simulink model "sim_sys2"  (R2013b)
settings: Solver=ode45  StartTime=0.0  StopTime=5000  RelTol=1e-3
undefined symbols (not defined in the file or in its folder): msdft_comb, resonator, sys_lib, twiddle_factors
libraries: xbsIndex_r4 x3996, casper_library_misc x310, xps_library x1
(part 2 of 46)

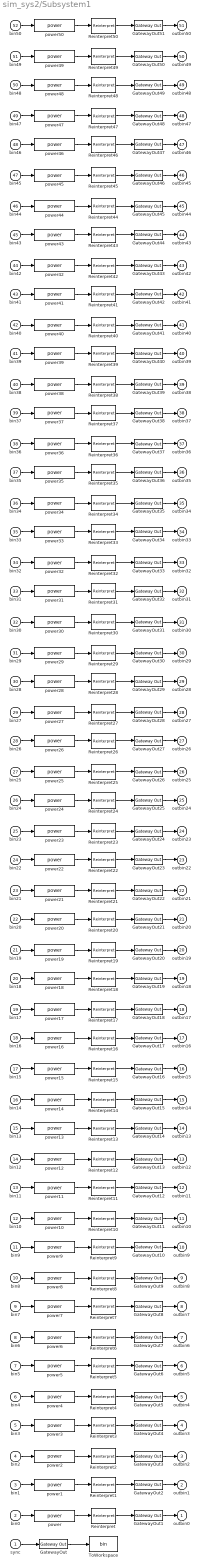
== system sim_sys2/Subsystem1 ==
  sync : Inport
  bin0 : Inport  Port=2
  bin1 : Inport  Port=3
  bin2 : Inport  Port=4
  bin3 : Inport  Port=5
  bin4 : Inport  Port=6
  bin5 : Inport  Port=7
  bin6 : Inport  Port=8
  bin7 : Inport  Port=9
  bin8 : Inport  Port=10
  bin9 : Inport  Port=11
  bin10 : Inport  Port=12
  bin11 : Inport  Port=13
  bin12 : Inport  Port=14
  bin13 : Inport  Port=15
  bin14 : Inport  Port=16
  bin15 : Inport  Port=17
  bin16 : Inport  Port=18
  bin17 : Inport  Port=19
  bin18 : Inport  Port=20
  bin19 : Inport  Port=21
  bin20 : Inport  Port=22
  bin21 : Inport  Port=23
  bin22 : Inport  Port=24
  bin23 : Inport  Port=25
  bin24 : Inport  Port=26
  bin25 : Inport  Port=27
  bin26 : Inport  Port=28
  bin27 : Inport  Port=29
  bin28 : Inport  Port=30
  bin29 : Inport  Port=31
  bin30 : Inport  Port=32
  bin31 : Inport  Port=33
  bin32 : Inport  Port=34
  bin33 : Inport  Port=35
  bin34 : Inport  Port=36
  bin35 : Inport  Port=37
  bin36 : Inport  Port=38
  bin37 : Inport  Port=39
  bin38 : Inport  Port=40
  bin39 : Inport  Port=41
  bin40 : Inport  Port=42
  bin41 : Inport  Port=43
  bin42 : Inport  Port=44
  bin43 : Inport  Port=45
  bin44 : Inport  Port=46
  bin45 : Inport  Port=47
  bin46 : Inport  Port=48
  bin47 : Inport  Port=49
  bin48 : Inport  Port=50
  bin49 : Inport  Port=51
  bin50 : Inport  Port=52
  GatewayOut{,1..51} (52 alike) : xbsIndex_r4/Gateway Out  inherit_from_input=on  hdl_port=on  timing_constraint=None  locs_specified=off  LOCs={}  UseAsDAC=off  DACChannel='1'  block_type=gatewayout
  Reinterpret{,1..50} (51 alike) : xbsIndex_r4/Reinterpret  force_arith_type=off  arith_type=Unsigned  force_bin_pt=on  bin_pt=0  block_type=reinterpret
  ToWorkspace : ToWorkspace  VariableName=bin  SampleTime=-1  SaveFormat=Timeseries
  power{,1..50} (51 alike) : casper_library_misc/power  BitWidth=40  add_latency=2  mult_latency=3
  outbin0 : Outport
  outbin1 : Outport  Port=2
  outbin2 : Outport  Port=3
  outbin3 : Outport  Port=4
  outbin4 : Outport  Port=5
  outbin5 : Outport  Port=6
  outbin6 : Outport  Port=7
  outbin7 : Outport  Port=8
  outbin8 : Outport  Port=9
  outbin9 : Outport  Port=10
  outbin10 : Outport  Port=11
  outbin11 : Outport  Port=12
  outbin12 : Outport  Port=13
  outbin13 : Outport  Port=14
  outbin14 : Outport  Port=15
  outbin15 : Outport  Port=16
  outbin16 : Outport  Port=17
  outbin17 : Outport  Port=18
  outbin18 : Outport  Port=19
  outbin19 : Outport  Port=20
  outbin20 : Outport  Port=21
  outbin21 : Outport  Port=22
  outbin22 : Outport  Port=23
  outbin23 : Outport  Port=24
  outbin24 : Outport  Port=25
  outbin25 : Outport  Port=26
  outbin26 : Outport  Port=27
  outbin27 : Outport  Port=28
  outbin28 : Outport  Port=29
  outbin29 : Outport  Port=30
  outbin30 : Outport  Port=31
  outbin31 : Outport  Port=32
  outbin32 : Outport  Port=33
  outbin33 : Outport  Port=34
  outbin34 : Outport  Port=35
  outbin35 : Outport  Port=36
  outbin36 : Outport  Port=37
  outbin37 : Outport  Port=38
  outbin38 : Outport  Port=39
  outbin39 : Outport  Port=40
  outbin40 : Outport  Port=41
  outbin41 : Outport  Port=42
  outbin42 : Outport  Port=43
  outbin43 : Outport  Port=44
  outbin44 : Outport  Port=45
  outbin45 : Outport  Port=46
  outbin46 : Outport  Port=47
  outbin47 : Outport  Port=48
  outbin48 : Outport  Port=49
  outbin49 : Outport  Port=50
  outbin50 : Outport  Port=51
  wires:
  GatewayOut51/1 -> outbin50/1
  Reinterpret50/1 -> GatewayOut51/1
  power50/1 -> Reinterpret50/1
  bin50/1 -> power50/1
  GatewayOut50/1 -> outbin49/1
  Reinterpret49/1 -> GatewayOut50/1
  power49/1 -> Reinterpret49/1
  bin49/1 -> power49/1
  GatewayOut49/1 -> outbin48/1
  Reinterpret48/1 -> GatewayOut49/1
  power48/1 -> Reinterpret48/1
  bin48/1 -> power48/1
  GatewayOut48/1 -> outbin47/1
  Reinterpret47/1 -> GatewayOut48/1
  power47/1 -> Reinterpret47/1
  bin47/1 -> power47/1
  GatewayOut47/1 -> outbin46/1
  Reinterpret46/1 -> GatewayOut47/1
  power46/1 -> Reinterpret46/1
  bin46/1 -> power46/1
  GatewayOut46/1 -> outbin45/1
  Reinterpret45/1 -> GatewayOut46/1
  power45/1 -> Reinterpret45/1
  bin45/1 -> power45/1
  GatewayOut45/1 -> outbin44/1
  Reinterpret44/1 -> GatewayOut45/1
  power44/1 -> Reinterpret44/1
  bin44/1 -> power44/1
  GatewayOut44/1 -> outbin43/1
  Reinterpret43/1 -> GatewayOut44/1
  power43/1 -> Reinterpret43/1
  bin43/1 -> power43/1
  GatewayOut43/1 -> outbin42/1
  Reinterpret42/1 -> GatewayOut43/1
  power42/1 -> Reinterpret42/1
  bin42/1 -> power42/1
  GatewayOut42/1 -> outbin41/1
  Reinterpret41/1 -> GatewayOut42/1
  power41/1 -> Reinterpret41/1
  bin41/1 -> power41/1
  GatewayOut41/1 -> outbin40/1
  Reinterpret40/1 -> GatewayOut41/1
  power40/1 -> Reinterpret40/1
  bin40/1 -> power40/1
  GatewayOut40/1 -> outbin39/1
  Reinterpret39/1 -> GatewayOut40/1
  power39/1 -> Reinterpret39/1
  bin39/1 -> power39/1
  GatewayOut39/1 -> outbin38/1
  Reinterpret38/1 -> GatewayOut39/1
  power38/1 -> Reinterpret38/1
  bin38/1 -> power38/1
  GatewayOut38/1 -> outbin37/1
  Reinterpret37/1 -> GatewayOut38/1
  power37/1 -> Reinterpret37/1
  bin37/1 -> power37/1
  GatewayOut37/1 -> outbin36/1
  Reinterpret36/1 -> GatewayOut37/1
  power36/1 -> Reinterpret36/1
  bin36/1 -> power36/1
  GatewayOut36/1 -> outbin35/1
  Reinterpret35/1 -> GatewayOut36/1
  power35/1 -> Reinterpret35/1
  bin35/1 -> power35/1
  GatewayOut35/1 -> outbin34/1
  Reinterpret34/1 -> GatewayOut35/1
  power34/1 -> Reinterpret34/1
  bin34/1 -> power34/1
  GatewayOut34/1 -> outbin33/1
  Reinterpret33/1 -> GatewayOut34/1
  power33/1 -> Reinterpret33/1
  bin33/1 -> power33/1
  GatewayOut33/1 -> outbin32/1
  Reinterpret32/1 -> GatewayOut33/1
  power32/1 -> Reinterpret32/1
  bin32/1 -> power32/1
  GatewayOut32/1 -> outbin31/1
  Reinterpret31/1 -> GatewayOut32/1
  power31/1 -> Reinterpret31/1
  bin31/1 -> power31/1
  GatewayOut31/1 -> outbin30/1
  Reinterpret30/1 -> GatewayOut31/1
  power30/1 -> Reinterpret30/1
  bin30/1 -> power30/1
  GatewayOut30/1 -> outbin29/1
  Reinterpret29/1 -> GatewayOut30/1
  power29/1 -> Reinterpret29/1
  bin29/1 -> power29/1
  GatewayOut29/1 -> outbin28/1
  Reinterpret28/1 -> GatewayOut29/1
  power28/1 -> Reinterpret28/1
  bin28/1 -> power28/1
  GatewayOut28/1 -> outbin27/1
  Reinterpret27/1 -> GatewayOut28/1
  power27/1 -> Reinterpret27/1
  bin27/1 -> power27/1
  GatewayOut27/1 -> outbin26/1
  Reinterpret26/1 -> GatewayOut27/1
  power26/1 -> Reinterpret26/1
  bin26/1 -> power26/1
  GatewayOut26/1 -> outbin25/1
  Reinterpret25/1 -> GatewayOut26/1
  power25/1 -> Reinterpret25/1
  bin25/1 -> power25/1
  GatewayOut25/1 -> outbin24/1
  Reinterpret24/1 -> GatewayOut25/1
  power24/1 -> Reinterpret24/1
  bin24/1 -> power24/1
  GatewayOut24/1 -> outbin23/1
  Reinterpret23/1 -> GatewayOut24/1
  power23/1 -> Reinterpret23/1
  bin23/1 -> power23/1
  GatewayOut23/1 -> outbin22/1
  Reinterpret22/1 -> GatewayOut23/1
  power22/1 -> Reinterpret22/1
  bin22/1 -> power22/1
  GatewayOut22/1 -> outbin21/1
  Reinterpret21/1 -> GatewayOut22/1
  power21/1 -> Reinterpret21/1
  bin21/1 -> power21/1
  GatewayOut21/1 -> outbin20/1
  Reinterpret20/1 -> GatewayOut21/1
  power20/1 -> Reinterpret20/1
  bin20/1 -> power20/1
  GatewayOut20/1 -> outbin19/1
  Reinterpret19/1 -> GatewayOut20/1
  power19/1 -> Reinterpret19/1
  bin19/1 -> power19/1
  GatewayOut19/1 -> outbin18/1
  Reinterpret18/1 -> GatewayOut19/1
  power18/1 -> Reinterpret18/1
  bin18/1 -> power18/1
  GatewayOut18/1 -> outbin17/1
  Reinterpret17/1 -> GatewayOut18/1
  power17/1 -> Reinterpret17/1
  bin17/1 -> power17/1
  GatewayOut17/1 -> outbin16/1
  Reinterpret16/1 -> GatewayOut17/1
  power16/1 -> Reinterpret16/1
  bin16/1 -> power16/1
  GatewayOut16/1 -> outbin15/1
  Reinterpret15/1 -> GatewayOut16/1
  power15/1 -> Reinterpret15/1
  bin15/1 -> power15/1
  GatewayOut15/1 -> outbin14/1
  Reinterpret14/1 -> GatewayOut15/1
  power14/1 -> Reinterpret14/1
  bin14/1 -> power14/1
  GatewayOut14/1 -> outbin13/1
  Reinterpret13/1 -> GatewayOut14/1
  power13/1 -> Reinterpret13/1
  bin13/1 -> power13/1
  GatewayOut13/1 -> outbin12/1
  Reinterpret12/1 -> GatewayOut13/1
  power12/1 -> Reinterpret12/1
  bin12/1 -> power12/1
  GatewayOut12/1 -> outbin11/1
  Reinterpret11/1 -> GatewayOut12/1
  power11/1 -> Reinterpret11/1
  bin11/1 -> power11/1
  GatewayOut11/1 -> outbin10/1
  Reinterpret10/1 -> GatewayOut11/1
  power10/1 -> Reinterpret10/1
  bin10/1 -> power10/1
  GatewayOut10/1 -> outbin9/1
  Reinterpret9/1 -> GatewayOut10/1
  power9/1 -> Reinterpret9/1
  bin9/1 -> power9/1
  GatewayOut9/1 -> outbin8/1
  Reinterpret8/1 -> GatewayOut9/1
  power8/1 -> Reinterpret8/1
  bin8/1 -> power8/1
  GatewayOut8/1 -> outbin7/1
  Reinterpret7/1 -> GatewayOut8/1
  power7/1 -> Reinterpret7/1
  bin7/1 -> power7/1
  GatewayOut7/1 -> outbin6/1
  Reinterpret6/1 -> GatewayOut7/1
  power6/1 -> Reinterpret6/1
  bin6/1 -> power6/1
  GatewayOut6/1 -> outbin5/1
  Reinterpret5/1 -> GatewayOut6/1
  power5/1 -> Reinterpret5/1
  bin5/1 -> power5/1
  GatewayOut5/1 -> outbin4/1
  Reinterpret4/1 -> GatewayOut5/1
  power4/1 -> Reinterpret4/1
  bin4/1 -> power4/1
  GatewayOut4/1 -> outbin3/1
  Reinterpret3/1 -> GatewayOut4/1
  power3/1 -> Reinterpret3/1
  bin3/1 -> power3/1
  GatewayOut3/1 -> outbin2/1
  Reinterpret2/1 -> GatewayOut3/1
  power2/1 -> Reinterpret2/1
  bin2/1 -> power2/1
  GatewayOut2/1 -> outbin1/1
  Reinterpret1/1 -> GatewayOut2/1
  power1/1 -> Reinterpret1/1
  bin1/1 -> power1/1
  GatewayOut1/1 -> outbin0/1
  Reinterpret/1 -> GatewayOut1/1
  power/1 -> Reinterpret/1
  bin0/1 -> power/1
  GatewayOut/1 -> ToWorkspace/1
  sync/1 -> GatewayOut/1

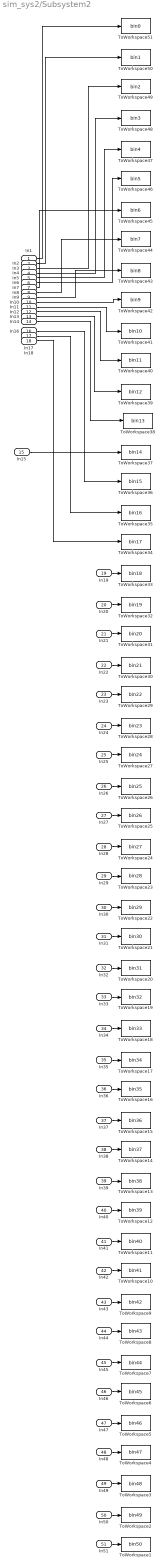
== system sim_sys2/Subsystem2 ==
  In1 : Inport
  In2 : Inport  Port=2
  In3 : Inport  Port=3
  In4 : Inport  Port=4
  In5 : Inport  Port=5
  In6 : Inport  Port=6
  In7 : Inport  Port=7
  In8 : Inport  Port=8
  In9 : Inport  Port=9
  In10 : Inport  Port=10
  In11 : Inport  Port=11
  In12 : Inport  Port=12
  In13 : Inport  Port=13
  In14 : Inport  Port=14
  In15 : Inport  Port=15
  In16 : Inport  Port=16
  In17 : Inport  Port=17
  In18 : Inport  Port=18
  In19 : Inport  Port=19
  In20 : Inport  Port=20
  In21 : Inport  Port=21
  In22 : Inport  Port=22
  In23 : Inport  Port=23
  In24 : Inport  Port=24
  In25 : Inport  Port=25
  In26 : Inport  Port=26
  In27 : Inport  Port=27
  In28 : Inport  Port=28
  In29 : Inport  Port=29
  In30 : Inport  Port=30
  In31 : Inport  Port=31
  In32 : Inport  Port=32
  In33 : Inport  Port=33
  In34 : Inport  Port=34
  In35 : Inport  Port=35
  In36 : Inport  Port=36
  In37 : Inport  Port=37
  In38 : Inport  Port=38
  In39 : Inport  Port=39
  In40 : Inport  Port=40
  In41 : Inport  Port=41
  In42 : Inport  Port=42
  In43 : Inport  Port=43
  In44 : Inport  Port=44
  In45 : Inport  Port=45
  In46 : Inport  Port=46
  In47 : Inport  Port=47
  In48 : Inport  Port=48
  In49 : Inport  Port=49
  In50 : Inport  Port=50
  In51 : Inport  Port=51
  ToWorkspace1 : ToWorkspace  VariableName=bin50  SampleTime=-1  SaveFormat=Timeseries
  ToWorkspace10 : ToWorkspace  VariableName=bin41  SampleTime=-1  SaveFormat=Timeseries
  ToWorkspace11 : ToWorkspace  VariableName=bin40  SampleTime=-1  SaveFormat=Timeseries
  ToWorkspace12 : ToWorkspace  VariableName=bin39  SampleTime=-1  SaveFormat=Timeseries
  ToWorkspace13 : ToWorkspace  VariableName=bin38  SampleTime=-1  SaveFormat=Timeseries
  ToWorkspace14 : ToWorkspace  VariableName=bin37  SampleTime=-1  SaveFormat=Timeseries
  ToWorkspace15 : ToWorkspace  VariableName=bin36  SampleTime=-1  SaveFormat=Timeseries
  ToWorkspace16 : ToWorkspace  VariableName=bin35  SampleTime=-1  SaveFormat=Timeseries
  ToWorkspace17 : ToWorkspace  VariableName=bin34  SampleTime=-1  SaveFormat=Timeseries
  ToWorkspace18 : ToWorkspace  VariableName=bin33  SampleTime=-1  SaveFormat=Timeseries
  ToWorkspace19 : ToWorkspace  VariableName=bin32  SampleTime=-1  SaveFormat=Timeseries
  ToWorkspace2 : ToWorkspace  VariableName=bin49  SampleTime=-1  SaveFormat=Timeseries
  ToWorkspace20 : ToWorkspace  VariableName=bin31  SampleTime=-1  SaveFormat=Timeseries
  ToWorkspace21 : ToWorkspace  VariableName=bin30  SampleTime=-1  SaveFormat=Timeseries
  ToWorkspace22 : ToWorkspace  VariableName=bin29  SampleTime=-1  SaveFormat=Timeseries
  ToWorkspace23 : ToWorkspace  VariableName=bin28  SampleTime=-1  SaveFormat=Timeseries
  ToWorkspace24 : ToWorkspace  VariableName=bin27  SampleTime=-1  SaveFormat=Timeseries
  ToWorkspace25 : ToWorkspace  VariableName=bin26  SampleTime=-1  SaveFormat=Timeseries
  ToWorkspace26 : ToWorkspace  VariableName=bin25  SampleTime=-1  SaveFormat=Timeseries
  ToWorkspace27 : ToWorkspace  VariableName=bin24  SampleTime=-1  SaveFormat=Timeseries
  ToWorkspace28 : ToWorkspace  VariableName=bin23  SampleTime=-1  SaveFormat=Timeseries
  ToWorkspace29 : ToWorkspace  VariableName=bin22  SampleTime=-1  SaveFormat=Timeseries
  ToWorkspace3 : ToWorkspace  VariableName=bin48  SampleTime=-1  SaveFormat=Timeseries
  ToWorkspace30 : ToWorkspace  VariableName=bin21  SampleTime=-1  SaveFormat=Timeseries
  ToWorkspace31 : ToWorkspace  VariableName=bin20  SampleTime=-1  SaveFormat=Timeseries
  ToWorkspace32 : ToWorkspace  VariableName=bin19  SampleTime=-1  SaveFormat=Timeseries
  ToWorkspace33 : ToWorkspace  VariableName=bin18  SampleTime=-1  SaveFormat=Timeseries
  ToWorkspace34 : ToWorkspace  VariableName=bin17  SampleTime=-1  SaveFormat=Timeseries
  ToWorkspace35 : ToWorkspace  VariableName=bin16  SampleTime=-1  SaveFormat=Timeseries
  ToWorkspace36 : ToWorkspace  VariableName=bin15  SampleTime=-1  SaveFormat=Timeseries
  ToWorkspace37 : ToWorkspace  VariableName=bin14  SampleTime=-1  SaveFormat=Timeseries
  ToWorkspace38 : ToWorkspace  VariableName=bin13  SampleTime=-1  SaveFormat=Timeseries
  ToWorkspace39 : ToWorkspace  VariableName=bin12  SampleTime=-1  SaveFormat=Timeseries
  ToWorkspace4 : ToWorkspace  VariableName=bin47  SampleTime=-1  SaveFormat=Timeseries
  ToWorkspace40 : ToWorkspace  VariableName=bin11  SampleTime=-1  SaveFormat=Timeseries
  ToWorkspace41 : ToWorkspace  VariableName=bin10  SampleTime=-1  SaveFormat=Timeseries
  ToWorkspace42 : ToWorkspace  VariableName=bin9  SampleTime=-1  SaveFormat=Timeseries
  ToWorkspace43 : ToWorkspace  VariableName=bin8  SampleTime=-1  SaveFormat=Timeseries
  ToWorkspace44 : ToWorkspace  VariableName=bin7  SampleTime=-1  SaveFormat=Timeseries
  ToWorkspace45 : ToWorkspace  VariableName=bin6  SampleTime=-1  SaveFormat=Timeseries
  ToWorkspace46 : ToWorkspace  VariableName=bin5  SampleTime=-1  SaveFormat=Timeseries
  ToWorkspace47 : ToWorkspace  VariableName=bin4  SampleTime=-1  SaveFormat=Timeseries
  ToWorkspace48 : ToWorkspace  VariableName=bin3  SampleTime=-1  SaveFormat=Timeseries
  ToWorkspace49 : ToWorkspace  VariableName=bin2  SampleTime=-1  SaveFormat=Timeseries
  ToWorkspace5 : ToWorkspace  VariableName=bin46  SampleTime=-1  SaveFormat=Timeseries
  ToWorkspace50 : ToWorkspace  VariableName=bin1  SampleTime=-1  SaveFormat=Timeseries
  ToWorkspace51 : ToWorkspace  VariableName=bin0  SampleTime=-1  SaveFormat=Timeseries
  ToWorkspace6 : ToWorkspace  VariableName=bin45  SampleTime=-1  SaveFormat=Timeseries
  ToWorkspace7 : ToWorkspace  VariableName=bin44  SampleTime=-1  SaveFormat=Timeseries
  ToWorkspace8 : ToWorkspace  VariableName=bin43  SampleTime=-1  SaveFormat=Timeseries
  ToWorkspace9 : ToWorkspace  VariableName=bin42  SampleTime=-1  SaveFormat=Timeseries
  wires:
  In2/1 -> ToWorkspace50/1
  In13/1 -> ToWorkspace39/1
  In5/1 -> ToWorkspace47/1
  In28/1 -> ToWorkspace24/1
  In35/1 -> ToWorkspace17/1
  In14/1 -> ToWorkspace38/1
  In36/1 -> ToWorkspace16/1
  In41/1 -> ToWorkspace11/1
  In26/1 -> ToWorkspace26/1
  In27/1 -> ToWorkspace25/1
  In12/1 -> ToWorkspace40/1
  In29/1 -> ToWorkspace23/1
  In34/1 -> ToWorkspace18/1
  In20/1 -> ToWorkspace32/1
  In37/1 -> ToWorkspace15/1
  In49/1 -> ToWorkspace3/1
  In40/1 -> ToWorkspace12/1
  In44/1 -> ToWorkspace8/1
  In39/1 -> ToWorkspace13/1
  In32/1 -> ToWorkspace20/1
  In50/1 -> ToWorkspace2/1
  In47/1 -> ToWorkspace5/1
  In30/1 -> ToWorkspace22/1
  In19/1 -> ToWorkspace33/1
  In42/1 -> ToWorkspace10/1
  In23/1 -> ToWorkspace29/1
  In43/1 -> ToWorkspace9/1
  In51/1 -> ToWorkspace1/1
  In46/1 -> ToWorkspace6/1
  In33/1 -> ToWorkspace19/1
  In22/1 -> ToWorkspace30/1
  In31/1 -> ToWorkspace21/1
  In38/1 -> ToWorkspace14/1
  In45/1 -> ToWorkspace7/1
  In24/1 -> ToWorkspace28/1
  In18/1 -> ToWorkspace34/1
  In9/1 -> ToWorkspace43/1
  In48/1 -> ToWorkspace4/1
  In10/1 -> ToWorkspace42/1
  In16/1 -> ToWorkspace36/1
  In15/1 -> ToWorkspace37/1
  In17/1 -> ToWorkspace35/1
  In6/1 -> ToWorkspace46/1
  In25/1 -> ToWorkspace27/1
  In21/1 -> ToWorkspace31/1
  In11/1 -> ToWorkspace41/1
  In1/1 -> ToWorkspace51/1
  In4/1 -> ToWorkspace48/1
  In3/1 -> ToWorkspace49/1
  In8/1 -> ToWorkspace44/1
  In7/1 -> ToWorkspace45/1

== system sim_sys2/Subsystem/msdft_comb ==
  sync : Inport
  rst : Inport  Port=2
  din : Inport  Port=3
  Constant : xbsIndex_r4/Constant  const=0  gui_display_data_type=Fixed-point  arith_type=Unsigned  n_bits=2*input_bitsize  bin_pt=0  preci_type=Single  exp_width=8  frac_width=24  explicit_period=on  period=1  equ=P=C  opselect=C  inp2=PCIN>>17  opr=+  inp1=P  carry=CIN  dbl_ovrd=off  block_type=constant
  Constant1 : xbsIndex_r4/Constant  const=0  gui_display_data_type=Fixed-point  arith_type=Unsigned  n_bits=2*(input_bitsize+1)  bin_pt=0  preci_type=Single  exp_width=8  frac_width=24  explicit_period=on  period=1  equ=P=C  opselect=C  inp2=PCIN>>17  opr=+  inp1=P  carry=CIN  dbl_ovrd=off  block_type=constant
  Delay : xbsIndex_r4/Delay  rst=off  infoeditControl=Selection of Reset will increase slice count due to use of real FFs and instead of SRLs  en=off  latency=2^fft_len  dbl_ovrd=off  reg_retiming=off  block_type=delay
  Delay1 : xbsIndex_r4/Delay  rst=off  infoeditControl=Selection of Reset will increase slice count due to use of real FFs and instead of SRLs  en=off  latency=2^fft_len-1  dbl_ovrd=off  reg_retiming=off  block_type=delay
  Mux : xbsIndex_r4/Mux  inputs=2  en=off  latency=0  precision=Full  arith_type=Unsigned  n_bits=16  bin_pt=14  quantization=Truncate  overflow=Wrap  dbl_ovrd=off  block_type=mux
  Mux1 : xbsIndex_r4/Mux  inputs=2  en=off  latency=0  precision=Full  arith_type=Unsigned  n_bits=16  bin_pt=14  quantization=Truncate  overflow=Wrap  dbl_ovrd=off  block_type=mux
  Register : xbsIndex_r4/Register  init=0  rst=on  en=on  dbl_ovrd=off  block_type=register
  complex_sub : Subsystem  mask(complex_sub){a_bitsize=input_bitsize, b_bitsize=input_bitsize, latency=0}
      mask init:
      | complex_sub_init(gcb, ...
      |             'a_bitsize', a_bitsize, ...
      |             'b_bitsize', b_bitsize, ...
      |             'latency', latency);
      settings: AttributesFormatString=latency=0
  dout : Outport
  wires:
  Delay1/1 -> Mux1/1
  Register/1 -> Delay1/1, Mux/1  "select"
  Mux/1 -> dout/1  "out"
  Mux1/1 -> complex_sub/2(b)
  Constant1/1 -> Mux/2
  Constant/1 -> Mux1/2
  Delay/1 -> Mux1/3
  complex_sub/1(Out1) -> Mux/3
  din/1 -> complex_sub/1("a "), Delay/1
  rst/1 -> Register/2
  sync/1 -> Register/1, Register/3

== system sim_sys2/Subsystem/resonator ==
  note: No estoy tan seguro
      | de este delay....
  din : Inport
  sync : Inport  Port=2
  rst : Inport  Port=3
  Delay{,1..2,4} (4 alike) : xbsIndex_r4/Delay  rst=off  infoeditControl=Selection of Reset will increase slice count due to use of real FFs and instead of SRLs  en=off  latency=1  dbl_ovrd=off  reg_retiming=off  block_type=delay
  Delay3 : xbsIndex_r4/Delay  rst=off  infoeditControl=Selection of Reset will increase slice count due to use of real FFs and instead of SRLs  en=off  latency=5  dbl_ovrd=off  reg_retiming=off  block_type=delay
  cmult : Subsystem  AncestorBlock=casper_library_multipliers/cmult  mask(cmult){n_bits_a=input_bitsize, bin_pt_a=input_frac, n_bits_b=twid_bitsize, bin_pt_b=twid_bitsize-2, n_bits_ab=input_bitsize+twid_bitsize+1, bin_pt_ab=input_frac+twid_bitsize-2, quantization=Truncate, overflow=Wrap, in_latency=0, mult_latency=3, add_latency=1, conv_latency=1, conjugated=off, async=off, pipelined_enable=on, multiplier_implementation=behavioral HDL}
      mask prompts: n_bits_a "Number of Bits 'a'"; bin_pt_a "Binary Point 'a'"; n_bits_b "Number of Bits 'b'"; bin_pt_b "Binary Point 'b'"; n_bits_ab "Number of Bits 'ab'"; bin_pt_ab "Binary Point 'ab'"; in_latency "Input latency"; mult_latency "Multiplier Latency"; add_latency "Adder Latency"; conv_latency "Convert latency"; conjugated "Conjugate"; async "asynchronous operation"; pipelined_enable "enable pipeline"; multiplier_implementation "Multiplier implementation"
      mask help:
      | Multiplies two complex numbers using 4 multipliers and 2 adders.
      | Conjugation is optional.
      mask init:
      | cmult_init(gcb, ...
      |     'n_bits_a',n_bits_a, ...
      |     'bin_pt_a',bin_pt_a, ...
      |     'n_bits_b',n_bits_b, ...
      |     'bin_pt_b',bin_pt_b, ...
      |     'n_bits_ab',n_bits_ab, ...
      |     'bin_pt_ab',bin_pt_ab, ...
      |     'quantization',quantization, ...
      |     'overflow', overflow, ...
      |     'in_latency', in_latency, ...
      |     'mult_latency', mult_latency, ...
      |     'add_latency', add_latency, ...
      |     'conv_latency', conv_latency, ...
      |     'conjugated', conjugated, ...
      |     'multiplier_implementation', multiplier_implementation, ...
      |     'async', async, ...
      |     'pipelined_enable', pipelined_enable);
      settings: AttributesFormatString=|
      | 11_9 * 15_13 ==> 27_22
      | Truncate, Wrap
      | Latency=0
      mask TypeOptions quantization: Truncate | Round  (unbiased: +/- Inf) | Round  (unbiased: Even Values)
      mask TypeOptions overflow: Wrap | Saturate | Flag as error
      mask TypeOptions multiplier_implementation: behavioral HDL | standard core | embedded multiplier core
  complex_conj : Subsystem  AncestorBlock=casper_library_misc/complex_conj  mask(complex_conj){n_inputs=1, n_bits=twid_bitsize, bin_pt=twid_bitsize-2, latency=1, overflow=Wrap}
      mask prompts: n_inputs "number simultaneous inputs"; n_bits "input bitwidth"; bin_pt "input binary point"; overflow "overflow strategy"
      mask help: Finds the complex conjugate of complex inputs.
      mask init:
      | complex_conj_init(gcb, ...
      |     'n_inputs', n_inputs, ...
      |     'n_bits', n_bits, ...
      |     'bin_pt', bin_pt, ...
      |     'latency', latency, ...
      |     'overflow', overflow);
      mask TypeOptions overflow: Wrap | Saturate | Flag as error
  complex_sum : Subsystem  mask(complex_sum){a_bitsize=input_bitsize+twid_bitsize+1, a_frac=input_frac+twid_bitsize-2, b_bitsize=res_bitsize, b_frac=input_frac+twid_bitsize-2, out_bitsize=res_bitsize, latency=add_lat}
      mask prompts: out_bitsize "output_bitsize"
      mask init:
      | complex_sum_init(gcb, ...
      |             'a_bitsize', a_bitsize, ...
      |             'a_frac', a_frac, ...
      |             'b_bitsize', b_bitsize, ...
      |             'b_frac', b_frac, ...
      |             'out_bitsize', out_bitsize, ...
      |             'latency', latency);
      settings: AttributesFormatString=latency=0
  twiddle : Subsystem  mask(msdft_twiddle_factors){fft_len=fft_len, bin_num=bin_number, twid_bitsize=twid_bitsize}
      mask prompts: fft_len "fft_len(2^)"; bin_num "bin number"; twid_bitsize "twiddle bitsize"
      mask init:
      | twid_msdft_init(gcb, ...
      |         'fft_len', fft_len, ...
      |         'bin_num', bin_num, ...
      |         'twid_bitsize', twid_bitsize)
      settings: AttributesFormatString=N=10, k=50
  Out1 : Outport
  twidd : Outport  Port=2
  wires:
  Delay4/1 -> twidd/1
  Delay3/1 -> Delay4/1
  Delay1/1 -> Delay3/1
  Delay2/1 -> complex_sum/2(b)
  complex_sum/1(dout) -> Out1/1, Delay2/1
  cmult/1(ab) -> complex_sum/1(a)
  Delay/1 -> cmult/1(a)
  complex_conj/1(z*) -> cmult/2(b)
  twiddle/1(dout) -> Delay1/1, complex_conj/1(z)
  din/1 -> Delay/1
  rst/1 -> twiddle/2(rst)
  sync/1 -> twiddle/1(sync)

== system sim_sys2/Subsystem/resonator1 ==
  note: No estoy tan seguro
      | de este delay....
  din : Inport
  sync : Inport  Port=2
  rst : Inport  Port=3
  Delay{,1..2,4} (4 alike) : xbsIndex_r4/Delay  rst=off  infoeditControl=Selection of Reset will increase slice count due to use of real FFs and instead of SRLs  en=off  latency=1  dbl_ovrd=off  reg_retiming=off  block_type=delay
  Delay3 : xbsIndex_r4/Delay  rst=off  infoeditControl=Selection of Reset will increase slice count due to use of real FFs and instead of SRLs  en=off  latency=5  dbl_ovrd=off  reg_retiming=off  block_type=delay
  cmult : Subsystem  AncestorBlock=casper_library_multipliers/cmult  mask(cmult){n_bits_a=input_bitsize, bin_pt_a=input_frac, n_bits_b=twid_bitsize, bin_pt_b=twid_bitsize-2, n_bits_ab=input_bitsize+twid_bitsize+1, bin_pt_ab=input_frac+twid_bitsize-2, quantization=Truncate, overflow=Wrap, in_latency=0, mult_latency=3, add_latency=1, conv_latency=1, conjugated=off, async=off, pipelined_enable=on, multiplier_implementation=behavioral HDL}
      mask prompts: n_bits_a "Number of Bits 'a'"; bin_pt_a "Binary Point 'a'"; n_bits_b "Number of Bits 'b'"; bin_pt_b "Binary Point 'b'"; n_bits_ab "Number of Bits 'ab'"; bin_pt_ab "Binary Point 'ab'"; in_latency "Input latency"; mult_latency "Multiplier Latency"; add_latency "Adder Latency"; conv_latency "Convert latency"; conjugated "Conjugate"; async "asynchronous operation"; pipelined_enable "enable pipeline"; multiplier_implementation "Multiplier implementation"
      mask help:
      | Multiplies two complex numbers using 4 multipliers and 2 adders.
      | Conjugation is optional.
      mask init: same as sim_sys2/Subsystem/resonator/cmult
      settings: AttributesFormatString=|
      | 11_9 * 15_13 ==> 27_22
      | Truncate, Wrap
      | Latency=0
      mask TypeOptions quantization: Truncate | Round  (unbiased: +/- Inf) | Round  (unbiased: Even Values)
      mask TypeOptions overflow: Wrap | Saturate | Flag as error
      mask TypeOptions multiplier_implementation: behavioral HDL | standard core | embedded multiplier core
  complex_conj : Subsystem  AncestorBlock=casper_library_misc/complex_conj  mask(complex_conj){n_inputs=1, n_bits=twid_bitsize, bin_pt=twid_bitsize-2, latency=1, overflow=Wrap}
      mask prompts: n_inputs "number simultaneous inputs"; n_bits "input bitwidth"; bin_pt "input binary point"; overflow "overflow strategy"
      mask help: Finds the complex conjugate of complex inputs.
      mask init:
      | complex_conj_init(gcb, ...
      |     'n_inputs', n_inputs, ...
      |     'n_bits', n_bits, ...
      |     'bin_pt', bin_pt, ...
      |     'latency', latency, ...
      |     'overflow', overflow);
      mask TypeOptions overflow: Wrap | Saturate | Flag as error
  complex_sum : Subsystem  mask(complex_sum){a_bitsize=input_bitsize+twid_bitsize+1, a_frac=input_frac+twid_bitsize-2, b_bitsize=res_bitsize, b_frac=input_frac+twid_bitsize-2, out_bitsize=res_bitsize, latency=add_lat}
      mask prompts: out_bitsize "output_bitsize"
      mask init: same as sim_sys2/Subsystem/resonator/complex_sum
      settings: AttributesFormatString=latency=0
  twiddle : Subsystem  mask(msdft_twiddle_factors){fft_len=fft_len, bin_num=bin_number, twid_bitsize=twid_bitsize}
      mask prompts: fft_len "fft_len(2^)"; bin_num "bin number"; twid_bitsize "twiddle bitsize"
      mask init:
      | twid_msdft_init(gcb, ...
      |         'fft_len', fft_len, ...
      |         'bin_num', bin_num, ...
      |         'twid_bitsize', twid_bitsize)
      settings: AttributesFormatString=N=10, k=51
  Out1 : Outport
  twidd : Outport  Port=2
  wires:
  Delay4/1 -> twidd/1
  Delay3/1 -> Delay4/1
  Delay1/1 -> Delay3/1
  Delay2/1 -> complex_sum/2(b)
  complex_sum/1(dout) -> Out1/1, Delay2/1
  cmult/1(ab) -> complex_sum/1(a)
  Delay/1 -> cmult/1(a)
  complex_conj/1(z*) -> cmult/2(b)
  twiddle/1(dout) -> Delay1/1, complex_conj/1(z)
  din/1 -> Delay/1
  rst/1 -> twiddle/2(rst)
  sync/1 -> twiddle/1(sync)

== system sim_sys2/Subsystem/resonator10 ==
  note: No estoy tan seguro
      | de este delay....
  din : Inport
  sync : Inport  Port=2
  rst : Inport  Port=3
  Delay{,1..2,4} (4 alike) : xbsIndex_r4/Delay  rst=off  infoeditControl=Selection of Reset will increase slice count due to use of real FFs and instead of SRLs  en=off  latency=1  dbl_ovrd=off  reg_retiming=off  block_type=delay
  Delay3 : xbsIndex_r4/Delay  rst=off  infoeditControl=Selection of Reset will increase slice count due to use of real FFs and instead of SRLs  en=off  latency=5  dbl_ovrd=off  reg_retiming=off  block_type=delay
  cmult : Subsystem  AncestorBlock=casper_library_multipliers/cmult  mask(cmult){n_bits_a=input_bitsize, bin_pt_a=input_frac, n_bits_b=twid_bitsize, bin_pt_b=twid_bitsize-2, n_bits_ab=input_bitsize+twid_bitsize+1, bin_pt_ab=input_frac+twid_bitsize-2, quantization=Truncate, overflow=Wrap, in_latency=0, mult_latency=3, add_latency=1, conv_latency=1, conjugated=off, async=off, pipelined_enable=on, multiplier_implementation=behavioral HDL}
      mask prompts: n_bits_a "Number of Bits 'a'"; bin_pt_a "Binary Point 'a'"; n_bits_b "Number of Bits 'b'"; bin_pt_b "Binary Point 'b'"; n_bits_ab "Number of Bits 'ab'"; bin_pt_ab "Binary Point 'ab'"; in_latency "Input latency"; mult_latency "Multiplier Latency"; add_latency "Adder Latency"; conv_latency "Convert latency"; conjugated "Conjugate"; async "asynchronous operation"; pipelined_enable "enable pipeline"; multiplier_implementation "Multiplier implementation"
      mask help:
      | Multiplies two complex numbers using 4 multipliers and 2 adders.
      | Conjugation is optional.
      mask init: same as sim_sys2/Subsystem/resonator/cmult
      settings: AttributesFormatString=|
      | 11_9 * 15_13 ==> 27_22
      | Truncate, Wrap
      | Latency=0
      mask TypeOptions quantization: Truncate | Round  (unbiased: +/- Inf) | Round  (unbiased: Even Values)
      mask TypeOptions overflow: Wrap | Saturate | Flag as error
      mask TypeOptions multiplier_implementation: behavioral HDL | standard core | embedded multiplier core
  complex_conj : Subsystem  AncestorBlock=casper_library_misc/complex_conj  mask(complex_conj){n_inputs=1, n_bits=twid_bitsize, bin_pt=twid_bitsize-2, latency=1, overflow=Wrap}
      mask prompts: n_inputs "number simultaneous inputs"; n_bits "input bitwidth"; bin_pt "input binary point"; overflow "overflow strategy"
      mask help: Finds the complex conjugate of complex inputs.
      mask init:
      | complex_conj_init(gcb, ...
      |     'n_inputs', n_inputs, ...
      |     'n_bits', n_bits, ...
      |     'bin_pt', bin_pt, ...
      |     'latency', latency, ...
      |     'overflow', overflow);
      mask TypeOptions overflow: Wrap | Saturate | Flag as error
  complex_sum : Subsystem  mask(complex_sum){a_bitsize=input_bitsize+twid_bitsize+1, a_frac=input_frac+twid_bitsize-2, b_bitsize=res_bitsize, b_frac=input_frac+twid_bitsize-2, out_bitsize=res_bitsize, latency=add_lat}
      mask prompts: out_bitsize "output_bitsize"
      mask init: same as sim_sys2/Subsystem/resonator/complex_sum
      settings: AttributesFormatString=latency=0
  twiddle : Subsystem  mask(msdft_twiddle_factors){fft_len=fft_len, bin_num=bin_number, twid_bitsize=twid_bitsize}
      mask prompts: fft_len "fft_len(2^)"; bin_num "bin number"; twid_bitsize "twiddle bitsize"
      mask init:
      | twid_msdft_init(gcb, ...
      |         'fft_len', fft_len, ...
      |         'bin_num', bin_num, ...
      |         'twid_bitsize', twid_bitsize)
      settings: AttributesFormatString=N=10, k=60
  Out1 : Outport
  twidd : Outport  Port=2
  wires:
  Delay4/1 -> twidd/1
  Delay3/1 -> Delay4/1
  Delay1/1 -> Delay3/1
  Delay2/1 -> complex_sum/2(b)
  complex_sum/1(dout) -> Out1/1, Delay2/1
  cmult/1(ab) -> complex_sum/1(a)
  Delay/1 -> cmult/1(a)
  complex_conj/1(z*) -> cmult/2(b)
  twiddle/1(dout) -> Delay1/1, complex_conj/1(z)
  din/1 -> Delay/1
  rst/1 -> twiddle/2(rst)
  sync/1 -> twiddle/1(sync)

== system sim_sys2/Subsystem/resonator11 ==
  note: No estoy tan seguro
      | de este delay....
  din : Inport
  sync : Inport  Port=2
  rst : Inport  Port=3
  Delay{,1..2,4} (4 alike) : xbsIndex_r4/Delay  rst=off  infoeditControl=Selection of Reset will increase slice count due to use of real FFs and instead of SRLs  en=off  latency=1  dbl_ovrd=off  reg_retiming=off  block_type=delay
  Delay3 : xbsIndex_r4/Delay  rst=off  infoeditControl=Selection of Reset will increase slice count due to use of real FFs and instead of SRLs  en=off  latency=5  dbl_ovrd=off  reg_retiming=off  block_type=delay
  cmult : Subsystem  AncestorBlock=casper_library_multipliers/cmult  mask(cmult){n_bits_a=input_bitsize, bin_pt_a=input_frac, n_bits_b=twid_bitsize, bin_pt_b=twid_bitsize-2, n_bits_ab=input_bitsize+twid_bitsize+1, bin_pt_ab=input_frac+twid_bitsize-2, quantization=Truncate, overflow=Wrap, in_latency=0, mult_latency=3, add_latency=1, conv_latency=1, conjugated=off, async=off, pipelined_enable=on, multiplier_implementation=behavioral HDL}
      mask prompts: n_bits_a "Number of Bits 'a'"; bin_pt_a "Binary Point 'a'"; n_bits_b "Number of Bits 'b'"; bin_pt_b "Binary Point 'b'"; n_bits_ab "Number of Bits 'ab'"; bin_pt_ab "Binary Point 'ab'"; in_latency "Input latency"; mult_latency "Multiplier Latency"; add_latency "Adder Latency"; conv_latency "Convert latency"; conjugated "Conjugate"; async "asynchronous operation"; pipelined_enable "enable pipeline"; multiplier_implementation "Multiplier implementation"
      mask help:
      | Multiplies two complex numbers using 4 multipliers and 2 adders.
      | Conjugation is optional.
      mask init: same as sim_sys2/Subsystem/resonator/cmult
      settings: AttributesFormatString=|
      | 11_9 * 15_13 ==> 27_22
      | Truncate, Wrap
      | Latency=0
      mask TypeOptions quantization: Truncate | Round  (unbiased: +/- Inf) | Round  (unbiased: Even Values)
      mask TypeOptions overflow: Wrap | Saturate | Flag as error
      mask TypeOptions multiplier_implementation: behavioral HDL | standard core | embedded multiplier core
  complex_conj : Subsystem  AncestorBlock=casper_library_misc/complex_conj  mask(complex_conj){n_inputs=1, n_bits=twid_bitsize, bin_pt=twid_bitsize-2, latency=1, overflow=Wrap}
      mask prompts: n_inputs "number simultaneous inputs"; n_bits "input bitwidth"; bin_pt "input binary point"; overflow "overflow strategy"
      mask help: Finds the complex conjugate of complex inputs.
      mask init:
      | complex_conj_init(gcb, ...
      |     'n_inputs', n_inputs, ...
      |     'n_bits', n_bits, ...
      |     'bin_pt', bin_pt, ...
      |     'latency', latency, ...
      |     'overflow', overflow);
      mask TypeOptions overflow: Wrap | Saturate | Flag as error
  complex_sum : Subsystem  mask(complex_sum){a_bitsize=input_bitsize+twid_bitsize+1, a_frac=input_frac+twid_bitsize-2, b_bitsize=res_bitsize, b_frac=input_frac+twid_bitsize-2, out_bitsize=res_bitsize, latency=add_lat}
      mask prompts: out_bitsize "output_bitsize"
      mask init: same as sim_sys2/Subsystem/resonator/complex_sum
      settings: AttributesFormatString=latency=0
  twiddle : Subsystem  mask(msdft_twiddle_factors){fft_len=fft_len, bin_num=bin_number, twid_bitsize=twid_bitsize}
      mask prompts: fft_len "fft_len(2^)"; bin_num "bin number"; twid_bitsize "twiddle bitsize"
      mask init:
      | twid_msdft_init(gcb, ...
      |         'fft_len', fft_len, ...
      |         'bin_num', bin_num, ...
      |         'twid_bitsize', twid_bitsize)
      settings: AttributesFormatString=N=10, k=61
  Out1 : Outport
  twidd : Outport  Port=2
  wires:
  Delay4/1 -> twidd/1
  Delay3/1 -> Delay4/1
  Delay1/1 -> Delay3/1
  Delay2/1 -> complex_sum/2(b)
  complex_sum/1(dout) -> Out1/1, Delay2/1
  cmult/1(ab) -> complex_sum/1(a)
  Delay/1 -> cmult/1(a)
  complex_conj/1(z*) -> cmult/2(b)
  twiddle/1(dout) -> Delay1/1, complex_conj/1(z)
  din/1 -> Delay/1
  rst/1 -> twiddle/2(rst)
  sync/1 -> twiddle/1(sync)

== system sim_sys2/Subsystem/resonator12 ==
  note: No estoy tan seguro
      | de este delay....
  din : Inport
  sync : Inport  Port=2
  rst : Inport  Port=3
  Delay{,1..2,4} (4 alike) : xbsIndex_r4/Delay  rst=off  infoeditControl=Selection of Reset will increase slice count due to use of real FFs and instead of SRLs  en=off  latency=1  dbl_ovrd=off  reg_retiming=off  block_type=delay
  Delay3 : xbsIndex_r4/Delay  rst=off  infoeditControl=Selection of Reset will increase slice count due to use of real FFs and instead of SRLs  en=off  latency=5  dbl_ovrd=off  reg_retiming=off  block_type=delay
  cmult : Subsystem  AncestorBlock=casper_library_multipliers/cmult  mask(cmult){n_bits_a=input_bitsize, bin_pt_a=input_frac, n_bits_b=twid_bitsize, bin_pt_b=twid_bitsize-2, n_bits_ab=input_bitsize+twid_bitsize+1, bin_pt_ab=input_frac+twid_bitsize-2, quantization=Truncate, overflow=Wrap, in_latency=0, mult_latency=3, add_latency=1, conv_latency=1, conjugated=off, async=off, pipelined_enable=on, multiplier_implementation=behavioral HDL}
      mask prompts: n_bits_a "Number of Bits 'a'"; bin_pt_a "Binary Point 'a'"; n_bits_b "Number of Bits 'b'"; bin_pt_b "Binary Point 'b'"; n_bits_ab "Number of Bits 'ab'"; bin_pt_ab "Binary Point 'ab'"; in_latency "Input latency"; mult_latency "Multiplier Latency"; add_latency "Adder Latency"; conv_latency "Convert latency"; conjugated "Conjugate"; async "asynchronous operation"; pipelined_enable "enable pipeline"; multiplier_implementation "Multiplier implementation"
      mask help:
      | Multiplies two complex numbers using 4 multipliers and 2 adders.
      | Conjugation is optional.
      mask init: same as sim_sys2/Subsystem/resonator/cmult
      settings: AttributesFormatString=|
      | 11_9 * 15_13 ==> 27_22
      | Truncate, Wrap
      | Latency=0
      mask TypeOptions quantization: Truncate | Round  (unbiased: +/- Inf) | Round  (unbiased: Even Values)
      mask TypeOptions overflow: Wrap | Saturate | Flag as error
      mask TypeOptions multiplier_implementation: behavioral HDL | standard core | embedded multiplier core
  complex_conj : Subsystem  AncestorBlock=casper_library_misc/complex_conj  mask(complex_conj){n_inputs=1, n_bits=twid_bitsize, bin_pt=twid_bitsize-2, latency=1, overflow=Wrap}
      mask prompts: n_inputs "number simultaneous inputs"; n_bits "input bitwidth"; bin_pt "input binary point"; overflow "overflow strategy"
      mask help: Finds the complex conjugate of complex inputs.
      mask init:
      | complex_conj_init(gcb, ...
      |     'n_inputs', n_inputs, ...
      |     'n_bits', n_bits, ...
      |     'bin_pt', bin_pt, ...
      |     'latency', latency, ...
      |     'overflow', overflow);
      mask TypeOptions overflow: Wrap | Saturate | Flag as error
  complex_sum : Subsystem  mask(complex_sum){a_bitsize=input_bitsize+twid_bitsize+1, a_frac=input_frac+twid_bitsize-2, b_bitsize=res_bitsize, b_frac=input_frac+twid_bitsize-2, out_bitsize=res_bitsize, latency=add_lat}
      mask prompts: out_bitsize "output_bitsize"
      mask init: same as sim_sys2/Subsystem/resonator/complex_sum
      settings: AttributesFormatString=latency=0
  twiddle : Subsystem  mask(msdft_twiddle_factors){fft_len=fft_len, bin_num=bin_number, twid_bitsize=twid_bitsize}
      mask prompts: fft_len "fft_len(2^)"; bin_num "bin number"; twid_bitsize "twiddle bitsize"
      mask init:
      | twid_msdft_init(gcb, ...
      |         'fft_len', fft_len, ...
      |         'bin_num', bin_num, ...
      |         'twid_bitsize', twid_bitsize)
      settings: AttributesFormatString=N=10, k=62
  Out1 : Outport
  twidd : Outport  Port=2
  wires:
  Delay4/1 -> twidd/1
  Delay3/1 -> Delay4/1
  Delay1/1 -> Delay3/1
  Delay2/1 -> complex_sum/2(b)
  complex_sum/1(dout) -> Out1/1, Delay2/1
  cmult/1(ab) -> complex_sum/1(a)
  Delay/1 -> cmult/1(a)
  complex_conj/1(z*) -> cmult/2(b)
  twiddle/1(dout) -> Delay1/1, complex_conj/1(z)
  din/1 -> Delay/1
  rst/1 -> twiddle/2(rst)
  sync/1 -> twiddle/1(sync)

== system sim_sys2/Subsystem/resonator13 ==
  note: No estoy tan seguro
      | de este delay....
  din : Inport
  sync : Inport  Port=2
  rst : Inport  Port=3
  Delay{,1..2,4} (4 alike) : xbsIndex_r4/Delay  rst=off  infoeditControl=Selection of Reset will increase slice count due to use of real FFs and instead of SRLs  en=off  latency=1  dbl_ovrd=off  reg_retiming=off  block_type=delay
  Delay3 : xbsIndex_r4/Delay  rst=off  infoeditControl=Selection of Reset will increase slice count due to use of real FFs and instead of SRLs  en=off  latency=5  dbl_ovrd=off  reg_retiming=off  block_type=delay
  cmult : Subsystem  AncestorBlock=casper_library_multipliers/cmult  mask(cmult){n_bits_a=input_bitsize, bin_pt_a=input_frac, n_bits_b=twid_bitsize, bin_pt_b=twid_bitsize-2, n_bits_ab=input_bitsize+twid_bitsize+1, bin_pt_ab=input_frac+twid_bitsize-2, quantization=Truncate, overflow=Wrap, in_latency=0, mult_latency=3, add_latency=1, conv_latency=1, conjugated=off, async=off, pipelined_enable=on, multiplier_implementation=behavioral HDL}
      mask prompts: n_bits_a "Number of Bits 'a'"; bin_pt_a "Binary Point 'a'"; n_bits_b "Number of Bits 'b'"; bin_pt_b "Binary Point 'b'"; n_bits_ab "Number of Bits 'ab'"; bin_pt_ab "Binary Point 'ab'"; in_latency "Input latency"; mult_latency "Multiplier Latency"; add_latency "Adder Latency"; conv_latency "Convert latency"; conjugated "Conjugate"; async "asynchronous operation"; pipelined_enable "enable pipeline"; multiplier_implementation "Multiplier implementation"
      mask help:
      | Multiplies two complex numbers using 4 multipliers and 2 adders.
      | Conjugation is optional.
      mask init: same as sim_sys2/Subsystem/resonator/cmult
      settings: AttributesFormatString=|
      | 11_9 * 15_13 ==> 27_22
      | Truncate, Wrap
      | Latency=0
      mask TypeOptions quantization: Truncate | Round  (unbiased: +/- Inf) | Round  (unbiased: Even Values)
      mask TypeOptions overflow: Wrap | Saturate | Flag as error
      mask TypeOptions multiplier_implementation: behavioral HDL | standard core | embedded multiplier core
  complex_conj : Subsystem  AncestorBlock=casper_library_misc/complex_conj  mask(complex_conj){n_inputs=1, n_bits=twid_bitsize, bin_pt=twid_bitsize-2, latency=1, overflow=Wrap}
      mask prompts: n_inputs "number simultaneous inputs"; n_bits "input bitwidth"; bin_pt "input binary point"; overflow "overflow strategy"
      mask help: Finds the complex conjugate of complex inputs.
      mask init:
      | complex_conj_init(gcb, ...
      |     'n_inputs', n_inputs, ...
      |     'n_bits', n_bits, ...
      |     'bin_pt', bin_pt, ...
      |     'latency', latency, ...
      |     'overflow', overflow);
      mask TypeOptions overflow: Wrap | Saturate | Flag as error
  complex_sum : Subsystem  mask(complex_sum){a_bitsize=input_bitsize+twid_bitsize+1, a_frac=input_frac+twid_bitsize-2, b_bitsize=res_bitsize, b_frac=input_frac+twid_bitsize-2, out_bitsize=res_bitsize, latency=add_lat}
      mask prompts: out_bitsize "output_bitsize"
      mask init: same as sim_sys2/Subsystem/resonator/complex_sum
      settings: AttributesFormatString=latency=0
  twiddle : Subsystem  mask(msdft_twiddle_factors){fft_len=fft_len, bin_num=bin_number, twid_bitsize=twid_bitsize}
      mask prompts: fft_len "fft_len(2^)"; bin_num "bin number"; twid_bitsize "twiddle bitsize"
      mask init:
      | twid_msdft_init(gcb, ...
      |         'fft_len', fft_len, ...
      |         'bin_num', bin_num, ...
      |         'twid_bitsize', twid_bitsize)
      settings: AttributesFormatString=N=10, k=63
  Out1 : Outport
  twidd : Outport  Port=2
  wires:
  Delay4/1 -> twidd/1
  Delay3/1 -> Delay4/1
  Delay1/1 -> Delay3/1
  Delay2/1 -> complex_sum/2(b)
  complex_sum/1(dout) -> Out1/1, Delay2/1
  cmult/1(ab) -> complex_sum/1(a)
  Delay/1 -> cmult/1(a)
  complex_conj/1(z*) -> cmult/2(b)
  twiddle/1(dout) -> Delay1/1, complex_conj/1(z)
  din/1 -> Delay/1
  rst/1 -> twiddle/2(rst)
  sync/1 -> twiddle/1(sync)

== system sim_sys2/Subsystem/resonator14 ==
  note: No estoy tan seguro
      | de este delay....
  din : Inport
  sync : Inport  Port=2
  rst : Inport  Port=3
  Delay{,1..2,4} (4 alike) : xbsIndex_r4/Delay  rst=off  infoeditControl=Selection of Reset will increase slice count due to use of real FFs and instead of SRLs  en=off  latency=1  dbl_ovrd=off  reg_retiming=off  block_type=delay
  Delay3 : xbsIndex_r4/Delay  rst=off  infoeditControl=Selection of Reset will increase slice count due to use of real FFs and instead of SRLs  en=off  latency=5  dbl_ovrd=off  reg_retiming=off  block_type=delay
  cmult : Subsystem  AncestorBlock=casper_library_multipliers/cmult  mask(cmult){n_bits_a=input_bitsize, bin_pt_a=input_frac, n_bits_b=twid_bitsize, bin_pt_b=twid_bitsize-2, n_bits_ab=input_bitsize+twid_bitsize+1, bin_pt_ab=input_frac+twid_bitsize-2, quantization=Truncate, overflow=Wrap, in_latency=0, mult_latency=3, add_latency=1, conv_latency=1, conjugated=off, async=off, pipelined_enable=on, multiplier_implementation=behavioral HDL}
      mask prompts: n_bits_a "Number of Bits 'a'"; bin_pt_a "Binary Point 'a'"; n_bits_b "Number of Bits 'b'"; bin_pt_b "Binary Point 'b'"; n_bits_ab "Number of Bits 'ab'"; bin_pt_ab "Binary Point 'ab'"; in_latency "Input latency"; mult_latency "Multiplier Latency"; add_latency "Adder Latency"; conv_latency "Convert latency"; conjugated "Conjugate"; async "asynchronous operation"; pipelined_enable "enable pipeline"; multiplier_implementation "Multiplier implementation"
      mask help:
      | Multiplies two complex numbers using 4 multipliers and 2 adders.
      | Conjugation is optional.
      mask init: same as sim_sys2/Subsystem/resonator/cmult
      settings: AttributesFormatString=|
      | 11_9 * 15_13 ==> 27_22
      | Truncate, Wrap
      | Latency=0
      mask TypeOptions quantization: Truncate | Round  (unbiased: +/- Inf) | Round  (unbiased: Even Values)
      mask TypeOptions overflow: Wrap | Saturate | Flag as error
      mask TypeOptions multiplier_implementation: behavioral HDL | standard core | embedded multiplier core
  complex_conj : Subsystem  AncestorBlock=casper_library_misc/complex_conj  mask(complex_conj){n_inputs=1, n_bits=twid_bitsize, bin_pt=twid_bitsize-2, latency=1, overflow=Wrap}
      mask prompts: n_inputs "number simultaneous inputs"; n_bits "input bitwidth"; bin_pt "input binary point"; overflow "overflow strategy"
      mask help: Finds the complex conjugate of complex inputs.
      mask init:
      | complex_conj_init(gcb, ...
      |     'n_inputs', n_inputs, ...
      |     'n_bits', n_bits, ...
      |     'bin_pt', bin_pt, ...
      |     'latency', latency, ...
      |     'overflow', overflow);
      mask TypeOptions overflow: Wrap | Saturate | Flag as error
  complex_sum : Subsystem  mask(complex_sum){a_bitsize=input_bitsize+twid_bitsize+1, a_frac=input_frac+twid_bitsize-2, b_bitsize=res_bitsize, b_frac=input_frac+twid_bitsize-2, out_bitsize=res_bitsize, latency=add_lat}
      mask prompts: out_bitsize "output_bitsize"
      mask init: same as sim_sys2/Subsystem/resonator/complex_sum
      settings: AttributesFormatString=latency=0
  twiddle : Subsystem  mask(msdft_twiddle_factors){fft_len=fft_len, bin_num=bin_number, twid_bitsize=twid_bitsize}
      mask prompts: fft_len "fft_len(2^)"; bin_num "bin number"; twid_bitsize "twiddle bitsize"
      mask init:
      | twid_msdft_init(gcb, ...
      |         'fft_len', fft_len, ...
      |         'bin_num', bin_num, ...
      |         'twid_bitsize', twid_bitsize)
      settings: AttributesFormatString=N=10, k=64
  Out1 : Outport
  twidd : Outport  Port=2
  wires:
  Delay4/1 -> twidd/1
  Delay3/1 -> Delay4/1
  Delay1/1 -> Delay3/1
  Delay2/1 -> complex_sum/2(b)
  complex_sum/1(dout) -> Out1/1, Delay2/1
  cmult/1(ab) -> complex_sum/1(a)
  Delay/1 -> cmult/1(a)
  complex_conj/1(z*) -> cmult/2(b)
  twiddle/1(dout) -> Delay1/1, complex_conj/1(z)
  din/1 -> Delay/1
  rst/1 -> twiddle/2(rst)
  sync/1 -> twiddle/1(sync)
